simulink model "quadcoptersVerification"  (R2021b)
settings: Solver=ode4  StartTime=0.0  StopTime=inf  FixedStep=sampleTime_base  RelTol=1e-3
InitFcn:
  | initial_condition_sim;
values from neighbouring files (symbols this model uses):
  inertia = inertia'    [initial_condition_sim.m]
  kd_att = kd_att'    [initial_condition_sim.m]
  kp_att = kp_att'    [initial_condition_sim.m]
  lb_pos = lb_pos'    [initial_condition_sim.m]
  lb_vel = lb_vel'    [initial_condition_sim.m]
  motor_init_con = states_omeges(14:17,:)    [initial_condition_sim.m]
  number = 6    [initial_condition_sim.m]
  sampleTime_base = 0.01    [initial_condition_sim.m]
  sampleTime_control = 0.01    [initial_condition_sim.m]
  ub_pos = ub_pos'    [initial_condition_sim.m]
  ub_vel = ub_vel'    [initial_condition_sim.m]
  vehicle_int_con = states_omeges(1:13,:)    [initial_condition_sim.m]
undefined symbols (not defined in the file or in its folder): aMax_h, aMax_v, cd_filter_pos, cd_filter_vel, cm, ct, euler_max, get_array_slice, gravity, lenArm, mass, T_re, thrust_max, vMax_h, vMax_v, yaw_rate_max
libraries: dspindex x7, aerolibanimutils x1
settings Model: Creator=huangjialei  LastModifiedBy=huangjlei
settings SolverCC: AlgebraicLoopSolver=TrustRegion

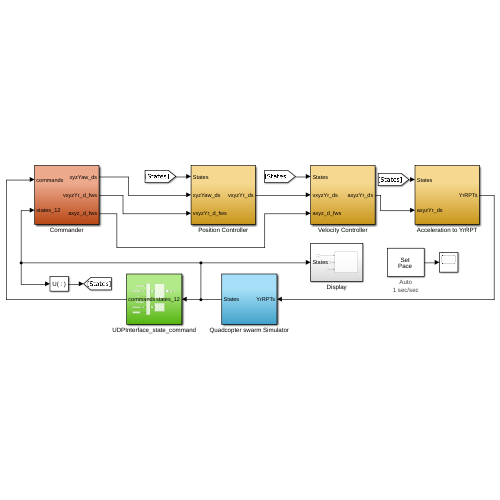
[thumbnail: Simulink's stored preview of the top-level diagram]
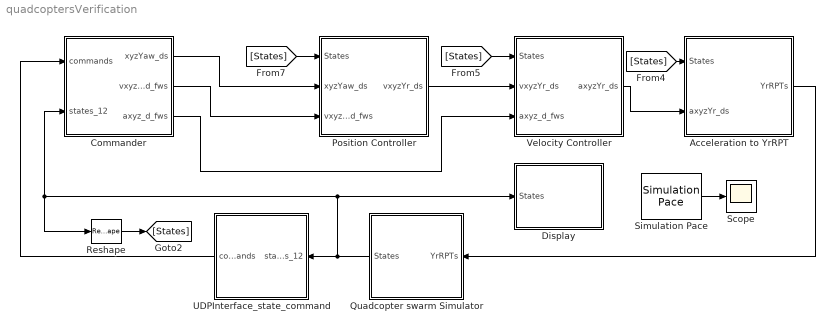
== system quadcoptersVerification ==
  Acceleration to YrRPT : Subsystem
  Commander : Subsystem
  Display : Subsystem
  Position Controller : Subsystem
  Quadcopter swarm Simulator : Subsystem
  Reshape : Reshape
  Scope : Scope
  Simulation Pace : aerolibanimutils/Simulation Pace  SimulationPace=1  SleepMode=Auto  OutputPaceError=on  SampleTime=sampleTime_base
  UDPInterface_state_command : Subsystem
  Velocity Controller : Subsystem
  wires:
  Commander/1(xyzYaw_ds) -> Position Controller/2(xyzYaw_ds)
  Commander/2(vxyzYr_d_fws) -> Position Controller/3(vxyzYr_d_fws)
  Simulation Pace/1 -> Scope/1
  Position Controller/1(vxyzYr_ds) -> Velocity Controller/2(vxyzYr_ds)
  Velocity Controller/1(axyzYr_ds) -> Acceleration to YrRPT/2(axyzYr_ds)
  Acceleration to YrRPT/1(YrRPTs) -> Quadcopter swarm Simulator/1(YrRPTs)
  [States] -> Acceleration to YrRPT/1(States)
  [States] -> Velocity Controller/1(States)
  [States] -> Position Controller/1(States)
  Commander/3(axyz_d_fws) -> Velocity Controller/3(axyz_d_fws)
  UDPInterface_state_command/1(commands) -> Commander/1(commands)
  Reshape/1 -> [States]
  Quadcopter swarm Simulator/1(States) -> UDPInterface_state_command/1(states_12), Commander/2(states_12), Reshape/1, Display/1(States)

== system quadcoptersVerification/Acceleration to YrRPT ==
  States : Inport
  axyzYr_ds : Inport  Port=2
  Selector : Selector  InputPortWidth=12*number  IndexOptions=Index vector (dialog)  Indices=10:12:12*number  OutputSizes=1
  Subsystem12 : Subsystem
  YrRPTs : Outport
  wires:
  States/1 -> Selector/1
  Selector/1 -> Subsystem12/2(yaws)
  Subsystem12/1(YrRPT) -> YrRPTs/1  "YrRPT"
  axyzYr_ds/1 -> Subsystem12/1(axyzYr_ds)

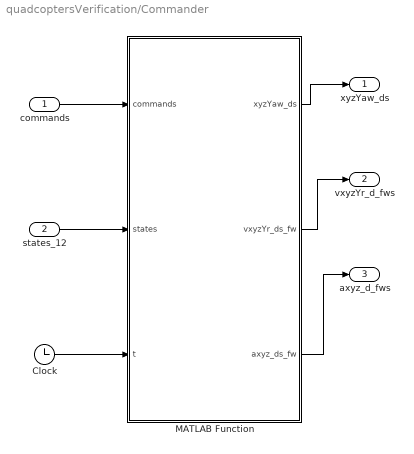
== system quadcoptersVerification/Commander ==
  commands : Inport
  states_12 : Inport  Port=2
  Clock : Clock
  MATLAB Function : MATLAB Function  TreatAsAtomicUnit=on  SystemSampleTime=sampleTime_control
  xyzYaw_ds : Outport
  vxyzYr_d_fws : Outport  Port=2
  axyz_d_fws : Outport  Port=3
  wires:
  Clock/1 -> MATLAB Function/3(t)
  MATLAB Function/2(vxyzYr_ds_fw) -> vxyzYr_d_fws/1
  MATLAB Function/1(xyzYaw_ds) -> xyzYaw_ds/1
  MATLAB Function/3(axyz_ds_fw) -> axyz_d_fws/1
  states_12/1 -> MATLAB Function/2(states)
  commands/1 -> MATLAB Function/1(commands)

== system quadcoptersVerification/Display ==
  States : Inport
  Clock : Clock
  Constant : Constant  Value=lenArm
  MATLAB Function : MATLAB Function  TreatAsAtomicUnit=on
  wires:
  Constant/1 -> MATLAB Function/2(lenArm)
  Clock/1 -> MATLAB Function/3(t)
  States/1 -> MATLAB Function/1(states)

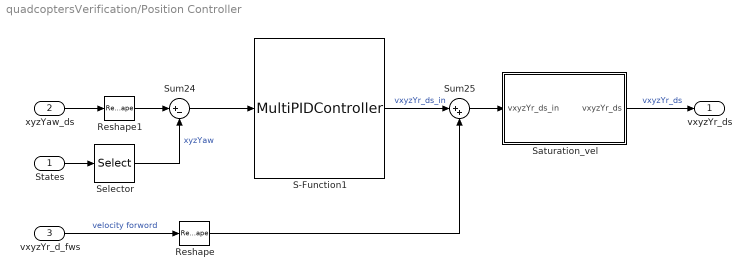
== system quadcoptersVerification/Position Controller ==
  States : Inport
  xyzYaw_ds : Inport  Port=2
  vxyzYr_d_fws : Inport  Port=3
  Reshape : Reshape
  Reshape1 : Reshape
  S-Function1 : S-Function  FunctionName=MultiPIDController  Parameters=sampleTime,number,width,enable_P,enable_I,enable_D,proportion,integral,derivative,c,enable_reset,lb,ub  SFunctionDeploymentMode=off  EnableBusSupport=off  mask{number=number, width=4, enable_P=on, enable_I=on, enable_D=on, proportion=[1,1,1,0], integral=[0,0,0,0], derivative=[0,0,3,0], c=cd_filter_pos, enable_reset=off, lb=lb_pos, ub=ub_pos, sampleTime=sampleTime_base}
      mask prompts: number "Number of input port"; width "Width of per input"; enable_P "Enable P"; enable_I "Enable I"; enable_D "Enable D"; c "Coefficient of low-pass filter in derivative part"; enable_reset "Rising edge reset of integral"; lb "Lower boundary of outputs"; ub "Upper boundary of outputs"; sampleTime "Sample time"
      mask Callback enable_P:
      | % disp(get_param(gcbh,'enable_P'))
      | % if strcmp(get_param(gcbh,'enable_P'), 'off')
      | %    disp(get_param(gcbh,'ParameterGroupVar'))
      | %
      | % end
  Saturation_vel : Subsystem
  Selector : Selector  InputPortWidth=12*number  IndexOptions=Index vector (dialog)  Indices=repmat([1,2,3,10],1,number) + reshape(repmat((0:number-1)*12,4,1),1,4*number)  OutputSizes=1
  Sum24 : Sum  Inputs=|+-
  Sum25 : Sum  Inputs=|++
  vxyzYr_ds : Outport
  wires:
  xyzYaw_ds/1 -> Reshape1/1
  States/1 -> Selector/1
  vxyzYr_d_fws/1 -> Reshape/1  "velocity forword"
  Sum24/1 -> S-Function1/1
  Selector/1 -> Sum24/2  "xyzYaw"
  S-Function1/1 -> Sum25/1  "vxyzYr_ds_in"
  Sum25/1 -> Saturation_vel/1(vxyzYr_ds_in)
  Saturation_vel/1(vxyzYr_ds) -> vxyzYr_ds/1  "vxyzYr_ds"
  Reshape/1 -> Sum25/2
  Reshape1/1 -> Sum24/1

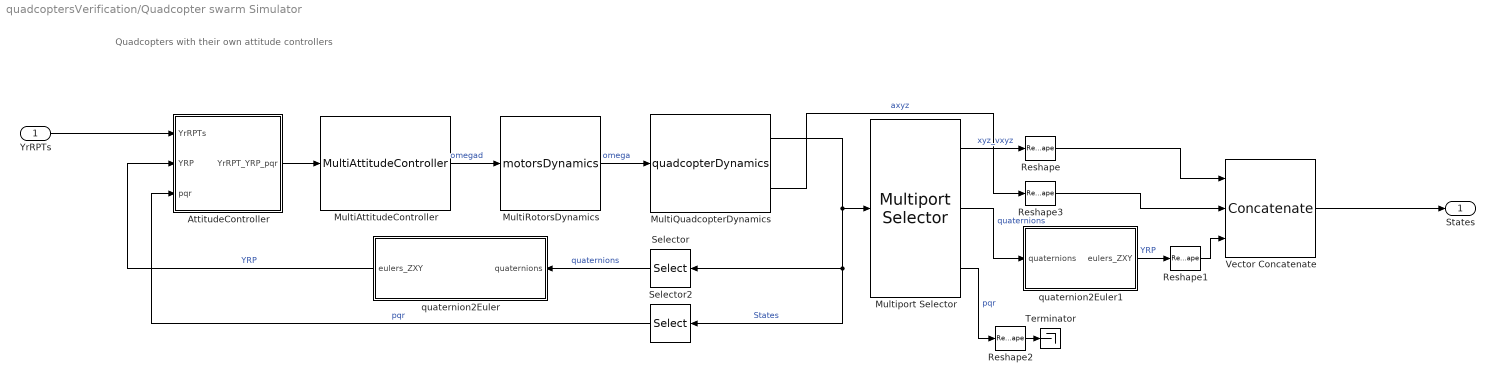
== system quadcoptersVerification/Quadcopter swarm Simulator ==
  note: Quadcopters with their own attitude controllers
  YrRPTs : Inport
  AttitudeController : Subsystem
  MultiAttitudeController : S-Function  FunctionName=MultiAttitudeController  Parameters=number_a,I_a,kp_a,kd_a,arm_length_a,ct_a,cm_a  SFunctionDeploymentMode=off  EnableBusSupport=off  mask{number_a=number+0, I_a=inertia, kp_a=kp_att, kd_a=kd_att, arm_length_a=lenArm, ct_a=ct, cm_a=cm}
      mask prompts: number_a "Number of quadcopters"; I_a "Moment of inertia"; kp_a "Coefficient of proportions"; kd_a "Coefficient of derivatives"; arm_length_a "Length of arm"; ct_a "Thrust coefficient of propeller"; cm_a "Moment coefficient of propeller"
      mask Display:
      | % number = get_param(gcbh,'number_a');
      | % for i = 1:str2num(number)
      | %    port_label('input', i, ['YrRPT_YRP_pqr',num2str(i)]);
      | % end
      | % for i = 1:str2num(number)
      | %    port_label('output', i, ['RPM_d',num2str(i)]);
      | % end
  MultiQuadcopterDynamics : S-Function  FunctionName=quadcopterDynamics  Parameters=number_q,mass_q,I_q,arm_length_q,ct_q,cm_q,conInit_q  SFunctionDeploymentMode=off  EnableBusSupport=off  mask{number_q=number+0, mass_q=mass, I_q=inertia, arm_length_q=lenArm, ct_q=ct, cm_q=cm, conInit_q=vehicle_int_con}
      mask prompts: number_q "Number of quadcopters"; mass_q "Mass"; I_q "Moment of inertia"; arm_length_q "Length of arm"; ct_q "Thrust coefficient of propeller"; cm_q "Moment coefficient of propeller"; conInit_q "Initial condition"
      mask Display:
      | number = get_param(gcbh,'number_q');
      | for i = 1:str2num(number)
      |    port_label('output', i, ['State',num2str(i)]);
      | end
      | for i = 1:str2num(number)
      |    port_label('input', i, ['RPM',num2str(i)]);
      | end
  MultiRotorsDynamics : S-Function  FunctionName=motorsDynamics  Parameters=number_m,K_m,conInit_m  SFunctionDeploymentMode=off  EnableBusSupport=off  mask{number_m=number+0, K_m=T_re, conInit_m=motor_init_con}
      mask prompts: number_m "Number of quadcopters"; K_m "Reciprocal of time constant"; conInit_m "Initial condition"
      mask Display:
      | number = get_param(gcbh,'number_m');
      | for i = 1:str2num(number)
      |    port_label('output', i, ['RPM',num2str(i)]);
      | end
      | for i = 1:str2num(number)
      |    port_label('input', i, ['RPM_d',num2str(i)]);
      | end
  Multiport Selector : dspindex/Multiport Selector  rowsOrCols=Rows  idxCellArray={ repmat(1:6,1,number) + reshape(repmat((0:number-1)*13,6,1),1,6*number),repmat(7:10,1,number) + reshape(repmat((0:number-1)*13,4,1),1,4*number), repmat(11:13,1,number) + reshape(repmat((0:number-1)*13,3,1),1,3*number)}  idxErrMode=Clip Index
  Reshape : Reshape  OutputDimensionality=Customize  OutputDimensions=[6,number]
  Reshape1 : Reshape  OutputDimensionality=Customize  OutputDimensions=[3,number]
  Reshape2 : Reshape  OutputDimensionality=Customize  OutputDimensions=[3,number]
  Reshape3 : Reshape  OutputDimensionality=Customize  OutputDimensions=[3,number]
  Selector : Selector  InputPortWidth=13*number  IndexOptions=Index vector (dialog)  Indices=repmat([7,8,9,10],1,number) + reshape(repmat((0:number-1)*13,4,1),1,4*number)  OutputSizes=1
  Selector2 : Selector  InputPortWidth=13*number  IndexOptions=Index vector (dialog)  Indices=repmat([11,12,13],1,number) + reshape(repmat((0:number-1)*13,3,1),1,3*number)  OutputSizes=1
  Terminator : Terminator
  Vector Concatenate : Concatenate  NumInputs=3  Mode=Multidimensional array
  quaternion2Euler : Subsystem
  quaternion2Euler1 : Subsystem
  States : Outport
  wires:
  YrRPTs/1 -> AttitudeController/1(YrRPTs)
  Selector/1 -> quaternion2Euler/1(quaternions)  "quaternions"
  quaternion2Euler/1(eulers_ZXY) -> AttitudeController/2(YRP)  "YRP"
  Selector2/1 -> AttitudeController/3(pqr)  "pqr"
  MultiAttitudeController/1 -> MultiRotorsDynamics/1  "omegad"
  MultiRotorsDynamics/1 -> MultiQuadcopterDynamics/1  "omega"
  MultiQuadcopterDynamics/1 -> Multiport Selector/1, Selector2/1, Selector/1  "States"
  Multiport Selector/2 -> quaternion2Euler1/1(quaternions)  "quaternions"
  Multiport Selector/1 -> Reshape/1  "xyz_vxyz"
  Reshape/1 -> Vector Concatenate/1
  quaternion2Euler1/1(eulers_ZXY) -> Reshape1/1  "YRP"
  Multiport Selector/3 -> Reshape2/1  "pqr"
  AttitudeController/1(YrRPT_YRP_pqr) -> MultiAttitudeController/1
  Vector Concatenate/1 -> States/1
  Reshape2/1 -> Terminator/1
  Reshape1/1 -> Vector Concatenate/3
  MultiQuadcopterDynamics/2 -> Reshape3/1  "axyz"
  Reshape3/1 -> Vector Concatenate/2

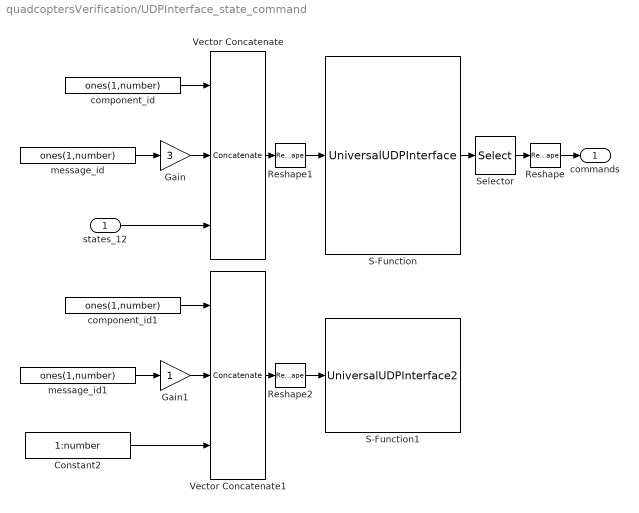
== system quadcoptersVerification/UDPInterface_state_command ==
  states_12 : Inport
  Constant2 : Constant  Value=1:number  VectorParams1D=off
  Gain : Gain  Gain=3
  Gain1 : Gain
  Reshape : Reshape  OutputDimensionality=Customize  OutputDimensions=[6,number]
  Reshape1 : Reshape
  Reshape2 : Reshape
  S-Function : S-Function  FunctionName=UniversalUDPInterface  Parameters=sampleTime,number,portTarget,portLocal,ipTarget,ipLocal,flagSend,flagRecv,inputPortWidth,outputPortWidth  SFunctionDeploymentMode=off  EnableBusSupport=off  mask{number=number, ipLocal=127.0.0.1, ipTarget=ones(1,number)*1, portTarget=20999, portLocal=21001, flagSend=on, flagRecv=on, inputPortWidth=14, outputPortWidth=9, sampleTime=sampleTime_control}
      mask prompts: number "Number of vehicles"; ipLocal "Local ip"; ipTarget "Target ip"; portTarget "Start port of target"; portLocal "Start port of local"; flagSend "Enable sender"; flagRecv "Enable receiver"; inputPortWidth "Width of input port"; outputPortWidth "Width of output port"; sampleTime "Sample time"
      mask help:
      | input port: componentId, messageId, msgData[0], msgData[1], ...
      | output port: systemId, numSequence, timeStamp,msgData[0], msgData[1], ...
  S-Function1 : S-Function  FunctionName=UniversalUDPInterface2  Parameters=sampleTime,number,portTarget,portLocal,ipTarget,ipLocal,flagSend,flagRecv,inputPortWidth,outputPortWidth  SFunctionDeploymentMode=off  EnableBusSupport=off  mask{number=number, ipLocal=127.0.0.1, ipTarget=ones(1,number)*1, portTarget=19999, portLocal=22001, flagSend=on, flagRecv=off, inputPortWidth=3, outputPortWidth=9, sampleTime=sampleTime_control}
      mask prompts: number "Number of vehicles"; ipLocal "Local ip"; ipTarget "Target ip"; portTarget "Start port of target"; portLocal "Start port of local"; flagSend "Enable sender"; flagRecv "Enable receiver"; inputPortWidth "Width of input port"; outputPortWidth "Width of output port"; sampleTime "Sample time"
      mask help:
      | input port: componentId, messageId, msgData[0], msgData[1], ...
      | output port: systemId, numSequence, timeStamp,msgData[0], msgData[1], ...
  Selector : Selector  InputPortWidth=9*number  IndexOptions=Index vector (dialog)  Indices=get_array_slice(4:9, number, 9)  OutputSizes=1
  Vector Concatenate : Concatenate  NumInputs=3  Mode=Multidimensional array
  Vector Concatenate1 : Concatenate  NumInputs=3  Mode=Multidimensional array
  component_id : Constant  Value=ones(1,number)  VectorParams1D=off
  component_id1 : Constant  Value=ones(1,number)  VectorParams1D=off
  message_id : Constant  Value=ones(1,number)  VectorParams1D=off
  message_id1 : Constant  Value=ones(1,number)  VectorParams1D=off
  commands : Outport
  wires:
  Vector Concatenate/1 -> Reshape1/1
  Reshape1/1 -> S-Function/1
  component_id/1 -> Vector Concatenate/1
  message_id/1 -> Gain/1
  Gain/1 -> Vector Concatenate/2
  S-Function/1 -> Selector/1
  Gain1/1 -> Vector Concatenate1/2
  message_id1/1 -> Gain1/1
  Constant2/1 -> Vector Concatenate1/3
  component_id1/1 -> Vector Concatenate1/1
  Reshape2/1 -> S-Function1/1
  Vector Concatenate1/1 -> Reshape2/1
  states_12/1 -> Vector Concatenate/3
  Selector/1 -> Reshape/1
  Reshape/1 -> commands/1

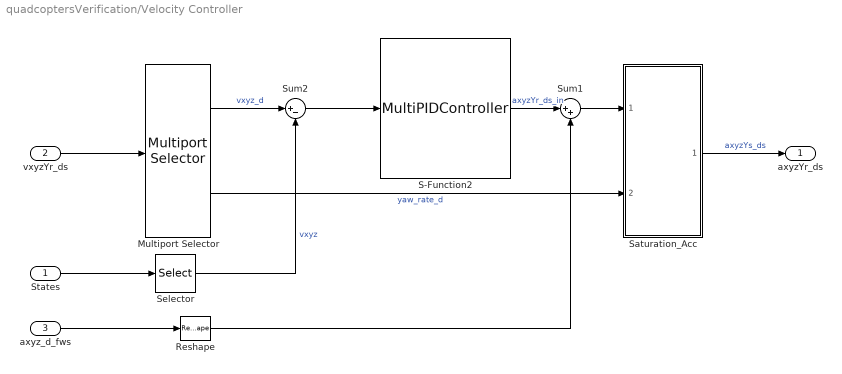
== system quadcoptersVerification/Velocity Controller ==
  States : Inport
  vxyzYr_ds : Inport  Port=2
  axyz_d_fws : Inport  Port=3
  Multiport Selector : dspindex/Multiport Selector  rowsOrCols=Rows  idxCellArray={ repmat([1,2,3],1,number) + reshape(repmat((0:number-1)*4,3,1),1,3*number),4:4:4*number}  idxErrMode=Clip Index
  Reshape : Reshape
  S-Function2 : S-Function  FunctionName=MultiPIDController  Parameters=sampleTime,number,width,enable_P,enable_I,enable_D,proportion,integral,derivative,c,enable_reset,lb,ub  SFunctionDeploymentMode=off  EnableBusSupport=off  mask{number=number+0, width=3, enable_P=on, enable_I=on, enable_D=on, proportion=[1.2,1.2,1], integral=[2,2,0.8], derivative=[0.3,0.3,0], c=cd_filter_vel, enable_reset=off, lb=lb_vel, ub=ub_vel, sampleTime=sampleTime_base}
      mask prompts: number "Number of input port"; width "Width of per input"; enable_P "Enable P"; enable_I "Enable I"; enable_D "Enable D"; c "Coefficient of low-pass filter in derivative part"; enable_reset "Rising edge reset of integral"; lb "Lower boundary of outputs"; ub "Upper boundary of outputs"; sampleTime "Sample time"
      mask Callback enable_P:
      | % disp(get_param(gcbh,'enable_P'))
      | % if strcmp(get_param(gcbh,'enable_P'), 'off')
      | %    disp(get_param(gcbh,'ParameterGroupVar'))
      | %
      | % end
  Saturation_Acc : Subsystem
  Selector : Selector  InputPortWidth=12*number  IndexOptions=Index vector (dialog)  Indices=repmat([4,5,6],1,number) + reshape(repmat((0:number-1)*12,3,1),1,3*number)  OutputSizes=1
  Sum1 : Sum  Inputs=|++
  Sum2 : Sum  Inputs=|+-
  axyzYr_ds : Outport
  wires:
  States/1 -> Selector/1
  Selector/1 -> Sum2/2  "vxyz"
  Sum2/1 -> S-Function2/1
  Multiport Selector/1 -> Sum2/1  "vxyz_d"
  Multiport Selector/2 -> Saturation_Acc/2(yaw_rates)  "yaw_rate_d"
  vxyzYr_ds/1 -> Multiport Selector/1
  Saturation_Acc/1(axyzYr_ds) -> axyzYr_ds/1  "axyzYs_ds"
  S-Function2/1 -> Sum1/1  "axyzYr_ds_in"
  Sum1/1 -> Saturation_Acc/1(axyz_d_in)
  axyz_d_fws/1 -> Reshape/1
  Reshape/1 -> Sum1/2

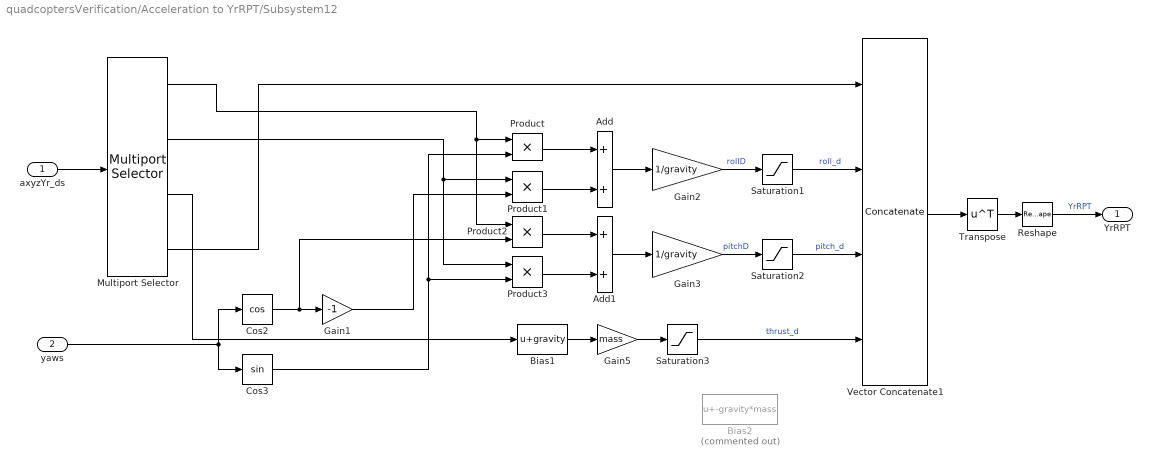
== system quadcoptersVerification/Acceleration to YrRPT/Subsystem12 ==
  axyzYr_ds : Inport
  yaws : Inport  Port=2
  Add : Sum
  Add1 : Sum
  Bias1 : Bias  Bias=gravity
  Bias2 : Bias  Commented=on  Bias=-gravity*mass
  Cos2 : Trigonometry  Operator=cos
  Cos3 : Trigonometry
  Gain1 : Gain  Gain=-1
  Gain2 : Gain  Gain=1/gravity
  Gain3 : Gain  Gain=1/gravity
  Gain5 : Gain  Gain=mass
  Multiport Selector : dspindex/Multiport Selector  rowsOrCols=Rows  idxCellArray={ 1:4:4*number,2:4:4*number, 3:4:4*number,4:4:4*number}  idxErrMode=Clip Index
  Product{,1..3} (4 alike) : Product
  Reshape : Reshape
  Saturation1 : Saturate  UpperLimit=euler_max  LowerLimit=-euler_max
  Saturation2 : Saturate  UpperLimit=euler_max  LowerLimit=-euler_max
  Saturation3 : Saturate  UpperLimit=thrust_max  LowerLimit=0
  Transpose : Math  Operator=transpose  SaturateOnIntegerOverflow=on
  Vector Concatenate1 : Concatenate  NumInputs=4  Mode=Multidimensional array  ConcatenateDimension=2
  YrRPT : Outport
  wires:
  Saturation3/1 -> Vector Concatenate1/4  "thrust_d"
  Saturation2/1 -> Vector Concatenate1/3  "pitch_d"
  Saturation1/1 -> Vector Concatenate1/2  "roll_d"
  Gain5/1 -> Saturation3/1
  Multiport Selector/4 -> Vector Concatenate1/1
  Reshape/1 -> YrRPT/1  "YrRPT"
  Gain2/1 -> Saturation1/1  "rollD"
  Add/1 -> Gain2/1
  Multiport Selector/1 -> Product/1, Product2/1
  Gain1/1 -> Product1/2
  Product/1 -> Add/1
  axyzYr_ds/1 -> Multiport Selector/1
  Product3/1 -> Add1/2
  Cos2/1 -> Gain1/1, Product2/2
  Product1/1 -> Add/2
  Multiport Selector/3 -> Bias1/1
  Gain3/1 -> Saturation2/1  "pitchD"
  Product2/1 -> Add1/1
  Multiport Selector/2 -> Product1/1, Product3/1
  Cos3/1 -> Product3/2, Product/2
  Add1/1 -> Gain3/1
  yaws/1 -> Cos2/1, Cos3/1
  Bias1/1 -> Gain5/1
  Vector Concatenate1/1 -> Transpose/1
  Transpose/1 -> Reshape/1

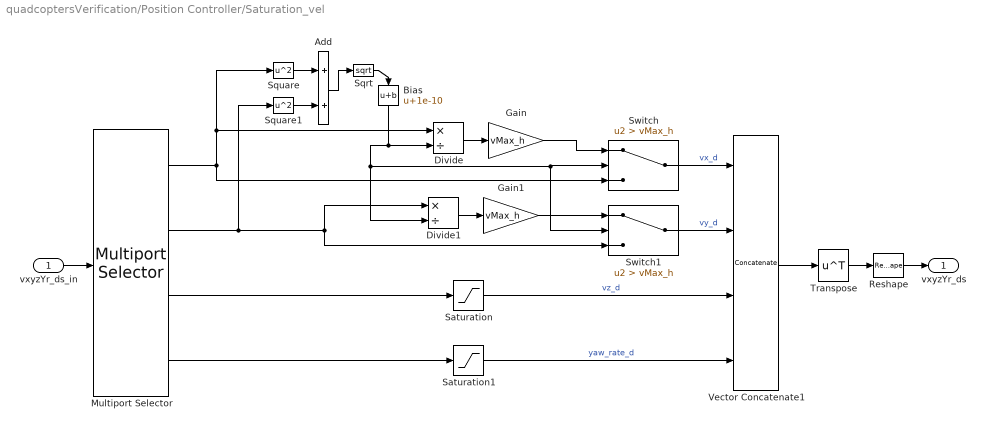
== system quadcoptersVerification/Position Controller/Saturation_vel ==
  vxyzYr_ds_in : Inport
  Add : Sum
  Bias : Bias  Bias=1e-10
  Divide : Product  Inputs=*/
  Divide1 : Product  Inputs=*/
  Gain : Gain  Gain=vMax_h
  Gain1 : Gain  Gain=vMax_h
  Multiport Selector : dspindex/Multiport Selector  rowsOrCols=Rows  idxCellArray={ 1:4:4*number,2:4:4*number, 3:4:4*number, 4:4:4*number }  idxErrMode=Clip Index
  Reshape : Reshape
  Saturation : Saturate  UpperLimit=vMax_v  LowerLimit=-vMax_v
  Saturation1 : Saturate  UpperLimit=yaw_rate_max  LowerLimit=-yaw_rate_max
  Sqrt : Sqrt  SaturateOnIntegerOverflow=on
  Square : Math  Operator=square  SaturateOnIntegerOverflow=on
  Square1 : Math  Operator=square  SaturateOnIntegerOverflow=on
  Switch : Switch  Criteria=u2 > Threshold  Threshold=vMax_h
  Switch1 : Switch  Criteria=u2 > Threshold  Threshold=vMax_h
  Transpose : Math  Operator=transpose  SaturateOnIntegerOverflow=on
  Vector Concatenate1 : Concatenate  NumInputs=4  Mode=Multidimensional array  ConcatenateDimension=2
  vxyzYr_ds : Outport
  wires:
  Switch/1 -> Vector Concatenate1/1  "vx_d"
  Multiport Selector/3 -> Saturation/1
  Gain/1 -> Switch/1
  Divide/1 -> Gain/1
  Multiport Selector/1 -> Square/1, Divide/1, Switch/3
  Add/1 -> Sqrt/1
  Square1/1 -> Add/2
  Square/1 -> Add/1
  vxyzYr_ds_in/1 -> Multiport Selector/1
  Multiport Selector/4 -> Saturation1/1
  Saturation1/1 -> Vector Concatenate1/4  "yaw_rate_d"
  Saturation/1 -> Vector Concatenate1/3  "vz_d"
  Sqrt/1 -> Bias/1
  Multiport Selector/2 -> Divide1/1, Switch1/3, Square1/1
  Divide1/1 -> Gain1/1
  Gain1/1 -> Switch1/1
  Switch1/1 -> Vector Concatenate1/2  "vy_d"
  Vector Concatenate1/1 -> Transpose/1
  Transpose/1 -> Reshape/1
  Reshape/1 -> vxyzYr_ds/1
  Bias/1 -> Divide/2, Divide1/2, Switch/2, Switch1/2

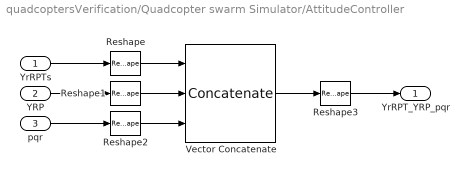
== system quadcoptersVerification/Quadcopter swarm Simulator/AttitudeController ==
  YrRPTs : Inport
  YRP : Inport  Port=2
  pqr : Inport  Port=3
  Reshape : Reshape  OutputDimensionality=Customize  OutputDimensions=[4,number]
  Reshape1 : Reshape  OutputDimensionality=Customize  OutputDimensions=[3,number]
  Reshape2 : Reshape  OutputDimensionality=Customize  OutputDimensions=[3,number]
  Reshape3 : Reshape
  Vector Concatenate : Concatenate  NumInputs=3  Mode=Multidimensional array
  YrRPT_YRP_pqr : Outport
  wires:
  YrRPTs/1 -> Reshape/1
  YRP/1 -> Reshape1/1
  pqr/1 -> Reshape2/1
  Reshape/1 -> Vector Concatenate/1
  Reshape1/1 -> Vector Concatenate/2
  Reshape2/1 -> Vector Concatenate/3
  Vector Concatenate/1 -> Reshape3/1
  Reshape3/1 -> YrRPT_YRP_pqr/1

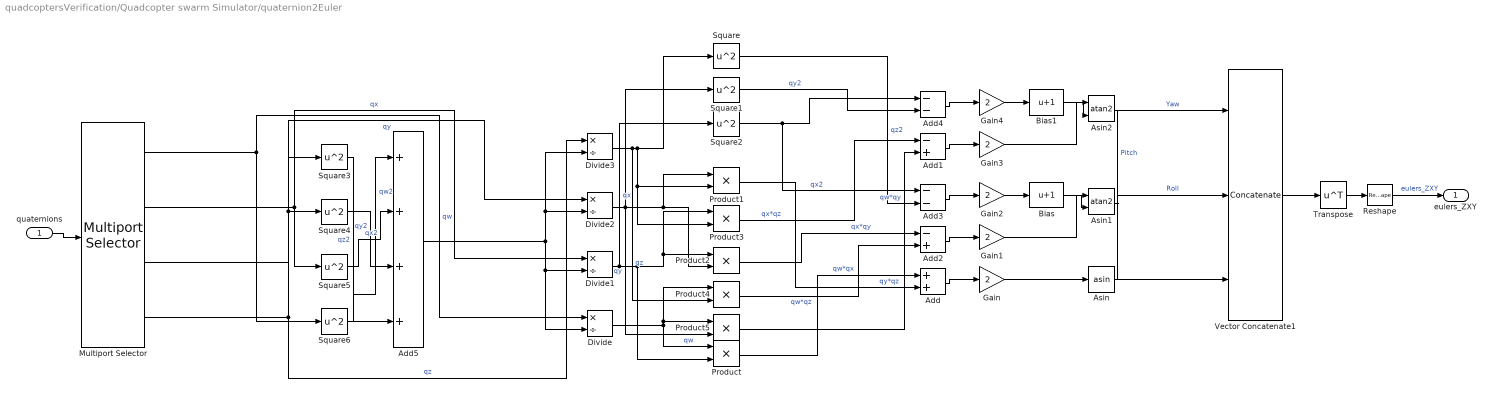
== system quadcoptersVerification/Quadcopter swarm Simulator/quaternion2Euler ==
  quaternions : Inport
  Add : Sum
  Add1 : Sum  Inputs=-+
  Add2 : Sum  Inputs=-+
  Add3 : Sum  Inputs=--
  Add4 : Sum  Inputs=--
  Add5 : Sum  Inputs=++++
  Asin : Trigonometry  Operator=asin
  Asin1 : Trigonometry  Operator=atan2
  Asin2 : Trigonometry  Operator=atan2
  Bias : Bias  Bias=1
  Bias1 : Bias  Bias=1
  Divide{,1..3} (4 alike) : Product  Inputs=*/
  Gain{,1..4} (5 alike) : Gain  Gain=2
  Multiport Selector : dspindex/Multiport Selector  rowsOrCols=Rows  idxCellArray={ 1:4:4*number,2:4:4*number, 3:4:4*number, 4:4:4*number }  idxErrMode=Clip Index
  Product{,1..5} (6 alike) : Product
  Reshape : Reshape
  Square{,1..6} (7 alike) : Math  Operator=square  SaturateOnIntegerOverflow=on
  Transpose : Math  Operator=transpose  SaturateOnIntegerOverflow=on
  Vector Concatenate1 : Concatenate  NumInputs=3  Mode=Multidimensional array  ConcatenateDimension=2
  eulers_ZXY : Outport
  wires:
  Multiport Selector/1 -> Divide/1, Square6/1  "qw"
  Add5/1 -> Divide1/2, Divide/2, Divide3/2, Divide2/2
  Square4/1 -> Add5/3  "qy2"
  Add/1 -> Gain/1
  quaternions/1 -> Multiport Selector/1
  Multiport Selector/4 -> Divide3/1, Square3/1  "qz"
  Product/1 -> Add/1  "qw*qx"
  Divide2/1 -> Product1/1, Product2/2, Product5/2, Square1/1  "qy"
  Reshape/1 -> eulers_ZXY/1  "eulers_ZXY"
  Product1/1 -> Add/2  "qy*qz"
  Divide1/1 -> Product3/1, Product2/1, Product/2, Square2/1  "qx"
  Square6/1 -> Add5/1  "qw2"
  Asin/1 -> Vector Concatenate1/2  "Roll"
  Square5/1 -> Add5/2  "qx2"
  Asin1/1 -> Vector Concatenate1/1  "Yaw"
  Product4/1 -> Add2/2  "qw*qz"
  Multiport Selector/2 -> Square5/1, Divide1/1  "qx"
  Product2/1 -> Add2/1  "qx*qy"
  Product3/1 -> Add1/1  "qx*qz"
  Gain/1 -> Asin/1
  Divide/1 -> Product5/1, Product4/1, Product/1  "qw"
  Gain3/1 -> Asin2/1
  Gain4/1 -> Bias1/1
  Divide3/1 -> Product3/2, Product1/2, Square/1, Product4/2  "qz"
  Square/1 -> Add3/2  "qz2"
  Add1/1 -> Gain3/1
  Bias1/1 -> Asin2/2
  Add2/1 -> Gain1/1
  Add4/1 -> Gain4/1
  Asin2/1 -> Vector Concatenate1/3  "Pitch"
  Multiport Selector/3 -> Divide2/1, Square4/1  "qy"
  Square3/1 -> Add5/4  "qz2"
  Square2/1 -> Add3/1, Add4/1  "qx2"
  Square1/1 -> Add4/2  "qy2"
  Vector Concatenate1/1 -> Transpose/1
  Bias/1 -> Asin1/2
  Gain2/1 -> Bias/1
  Add3/1 -> Gain2/1
  Gain1/1 -> Asin1/1
  Transpose/1 -> Reshape/1
  Product5/1 -> Add1/2  "qw*qy"

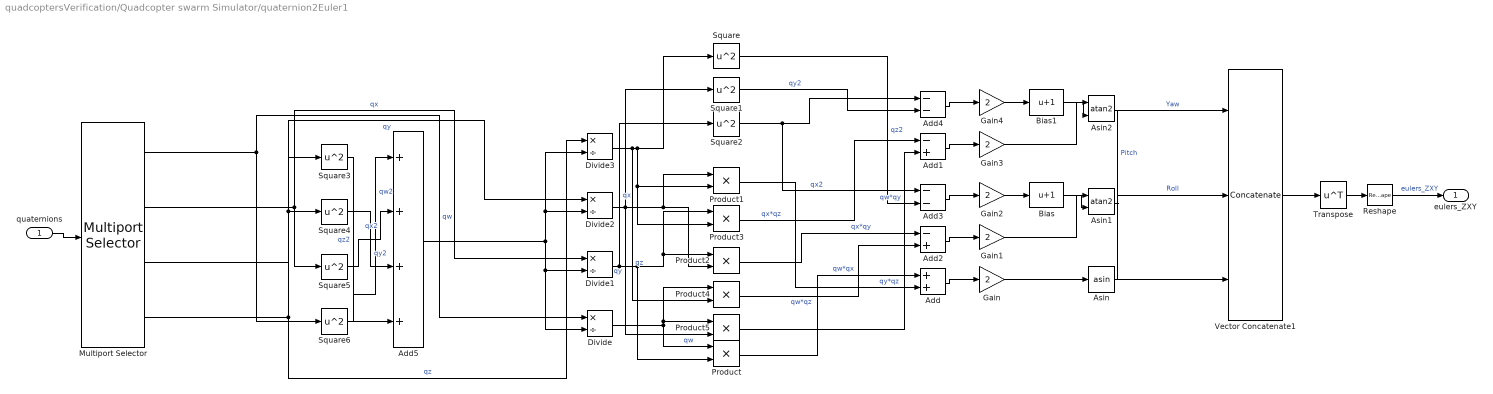
== system quadcoptersVerification/Quadcopter swarm Simulator/quaternion2Euler1 ==
  quaternions : Inport
  Add : Sum
  Add1 : Sum  Inputs=-+
  Add2 : Sum  Inputs=-+
  Add3 : Sum  Inputs=--
  Add4 : Sum  Inputs=--
  Add5 : Sum  Inputs=++++
  Asin : Trigonometry  Operator=asin
  Asin1 : Trigonometry  Operator=atan2
  Asin2 : Trigonometry  Operator=atan2
  Bias : Bias  Bias=1
  Bias1 : Bias  Bias=1
  Divide{,1..3} (4 alike) : Product  Inputs=*/
  Gain{,1..4} (5 alike) : Gain  Gain=2
  Multiport Selector : dspindex/Multiport Selector  rowsOrCols=Rows  idxCellArray={ 1:4:4*number,2:4:4*number, 3:4:4*number, 4:4:4*number }  idxErrMode=Clip Index
  Product{,1..5} (6 alike) : Product
  Reshape : Reshape
  Square{,1..6} (7 alike) : Math  Operator=square  SaturateOnIntegerOverflow=on
  Transpose : Math  Operator=transpose  SaturateOnIntegerOverflow=on
  Vector Concatenate1 : Concatenate  NumInputs=3  Mode=Multidimensional array  ConcatenateDimension=2
  eulers_ZXY : Outport
  wires:
  Product5/1 -> Add1/2  "qw*qy"
  Transpose/1 -> Reshape/1
  Gain1/1 -> Asin1/1
  Add3/1 -> Gain2/1
  Gain2/1 -> Bias/1
  Bias/1 -> Asin1/2
  Vector Concatenate1/1 -> Transpose/1
  Square1/1 -> Add4/2  "qy2"
  Square2/1 -> Add4/1, Add3/1  "qx2"
  Square3/1 -> Add5/4  "qz2"
  Multiport Selector/3 -> Square4/1, Divide2/1  "qy"
  Asin2/1 -> Vector Concatenate1/3  "Pitch"
  Add4/1 -> Gain4/1
  Add2/1 -> Gain1/1
  Bias1/1 -> Asin2/2
  Add1/1 -> Gain3/1
  Square/1 -> Add3/2  "qz2"
  Divide3/1 -> Product4/2, Square/1, Product1/2, Product3/2  "qz"
  Gain4/1 -> Bias1/1
  Gain3/1 -> Asin2/1
  Divide/1 -> Product/1, Product4/1, Product5/1  "qw"
  Gain/1 -> Asin/1
  Product3/1 -> Add1/1  "qx*qz"
  Product2/1 -> Add2/1  "qx*qy"
  Multiport Selector/2 -> Divide1/1, Square5/1  "qx"
  Product4/1 -> Add2/2  "qw*qz"
  Asin1/1 -> Vector Concatenate1/1  "Yaw"
  Square5/1 -> Add5/2  "qx2"
  Asin/1 -> Vector Concatenate1/2  "Roll"
  Square6/1 -> Add5/1  "qw2"
  Divide1/1 -> Square2/1, Product/2, Product2/1, Product3/1  "qx"
  Product1/1 -> Add/2  "qy*qz"
  Reshape/1 -> eulers_ZXY/1  "eulers_ZXY"
  Divide2/1 -> Square1/1, Product5/2, Product2/2, Product1/1  "qy"
  Product/1 -> Add/1  "qw*qx"
  Multiport Selector/4 -> Square3/1, Divide3/1  "qz"
  quaternions/1 -> Multiport Selector/1
  Add/1 -> Gain/1
  Square4/1 -> Add5/3  "qy2"
  Add5/1 -> Divide2/2, Divide3/2, Divide/2, Divide1/2
  Multiport Selector/1 -> Square6/1, Divide/1  "qw"

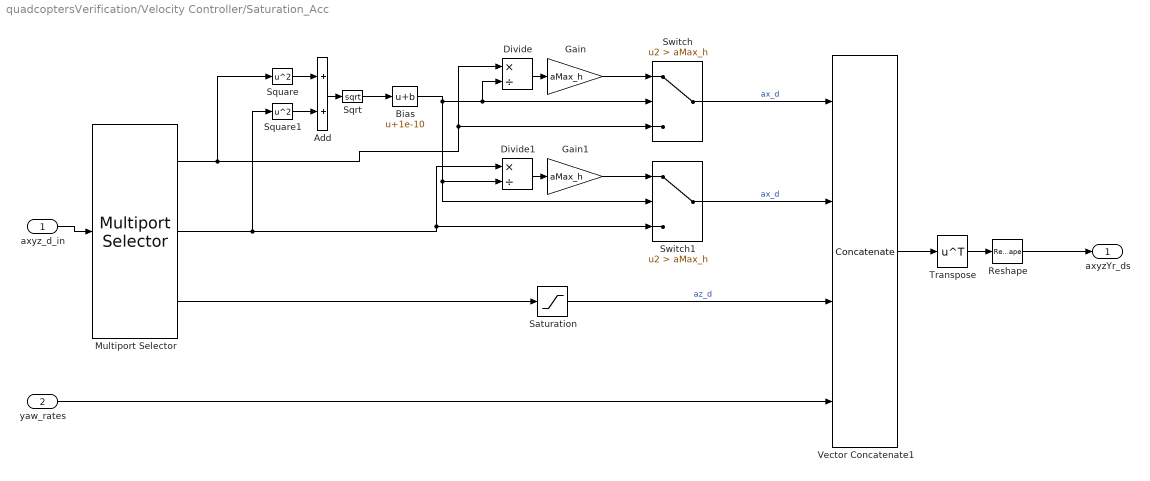
== system quadcoptersVerification/Velocity Controller/Saturation_Acc ==
  axyz_d_in : Inport
  yaw_rates : Inport  Port=2
  Add : Sum
  Bias : Bias  Bias=1e-10
  Divide : Product  Inputs=*/
  Divide1 : Product  Inputs=*/
  Gain : Gain  Gain=aMax_h
  Gain1 : Gain  Gain=aMax_h
  Multiport Selector : dspindex/Multiport Selector  rowsOrCols=Rows  idxCellArray={ 1:3:3*number,2:3:3*number, 3:3:3*number}  idxErrMode=Clip Index
  Reshape : Reshape
  Saturation : Saturate  UpperLimit=aMax_v  LowerLimit=-aMax_v
  Sqrt : Sqrt  SaturateOnIntegerOverflow=on
  Square : Math  Operator=square  SaturateOnIntegerOverflow=on
  Square1 : Math  Operator=square  SaturateOnIntegerOverflow=on
  Switch : Switch  Criteria=u2 > Threshold  Threshold=aMax_h
  Switch1 : Switch  Criteria=u2 > Threshold  Threshold=aMax_h
  Transpose : Math  Operator=transpose  SaturateOnIntegerOverflow=on
  Vector Concatenate1 : Concatenate  NumInputs=4  Mode=Multidimensional array  ConcatenateDimension=2
  axyzYr_ds : Outport
  wires:
  Switch/1 -> Vector Concatenate1/1  "ax_d"
  Saturation/1 -> Vector Concatenate1/3  "az_d"
  Reshape/1 -> axyzYr_ds/1
  Multiport Selector/3 -> Saturation/1
  Gain/1 -> Switch/1
  Divide/1 -> Gain/1
  Multiport Selector/1 -> Switch/3, Divide/1, Square/1
  Add/1 -> Sqrt/1
  Square1/1 -> Add/2
  Square/1 -> Add/1
  axyz_d_in/1 -> Multiport Selector/1
  Sqrt/1 -> Bias/1
  Multiport Selector/2 -> Switch1/3, Divide1/1, Square1/1
  Divide1/1 -> Gain1/1
  Gain1/1 -> Switch1/1
  Switch1/1 -> Vector Concatenate1/2  "ax_d"
  Transpose/1 -> Reshape/1
  Vector Concatenate1/1 -> Transpose/1
  yaw_rates/1 -> Vector Concatenate1/4
  Bias/1 -> Switch/2, Divide/2, Switch1/2, Divide1/2

== matlab function quadcoptersVerification/Commander/MATLAB Function ==
  settings: updateMethod=DISCRETE
  data: commands input; xyzYaw_ds output; states input; t input; vxyzYr_ds_fw output; axyz_ds_fw output
function [xyzYaw_ds, vxyzYr_ds_fw, axyz_ds_fw] = commander(commands, states,t)
persistent states_save  message_Ids_former t_start_Circle t_trigger v_save vx_save vy_save
number = size(states,2);
if isempty(states_save) || t < 0.1
    states_save = states;
    message_Ids_former = zeros(1,number)-1;
end
xyz_s = states(1:3,:);
% vxyz_s = states(4:6,:);
% axyz_s = states(7:9,:);
yrp_s = states(10:12,:);

xyzYaw_ds = [xyz_s;yrp_s(1,:)];
vxyzYr_ds_fw = zeros(4,number);
axyz_ds_fw   = zeros(3,number);



component_ids = commands(1,:);
message_ids = commands(2,:);
msgs = commands(3:6,:);

COMMAND_TYPE = 0;

Arming = 1;
Takeoff = 2;
Hover = 3;
Land = 4;
Position_control = 5;
Velocity_control = 6;
Velocity_horizontal_control = 7;
Acceleration_control = 8;

for id = 1:number
    component_id = component_ids(id);
    if component_id == COMMAND_TYPE
        message_id = message_ids(id);
        message_id_former = message_Ids_former(id);
        msg = msgs(:,id);
        switch message_id
            case Takeoff
                if message_id_former ~= message_id
%                     str = sprintf("UAV %d takeoff.",id);
%                     disp(str);
%                     disp(str);
                    fprintf("UAV %d takeoff.\n",int16(id));
                    states_save(:,id) = states(:,id);
                end
                xyzYaw_ds(:,id) = states_save([1,2,3,10],id);
                xyzYaw_ds(3,id) = msg(1);
            case Hover
                if message_id_former ~= message_id
%                     disp(['UAV ',num2str(id),' hover.']);
                    states_save(:,id) = states(:,id);
                end
                xyzYaw_ds(:,id) = states_save([1,2,3,10],id);
            case Land
                if message_id_former ~= message_id
%                     disp(['UAV ',num2str(id),' land.']);
                    states_save(:,id) = states(:,id);
                end
                xyzYaw_ds(:,id) = states_save([1,2,3,10],id);
                xyzYaw_ds(3,id) = msg(1);
            case Position_control
                if message_id_former ~= message_id
%                     disp(['UAV ',num2str(id),' position control.']);
                end
                xyzYaw_ds(:,id) = msg;
            case Velocity_control
                if message_id_former ~= message_id
%                     disp(['UAV ',num2str(id),' velocity control.']);
                end
                vxyzYr_ds_fw(:,id) = msg;
            case Velocity_horizontal_control
                if message_id_former ~= message_id
%                     disp(['UAV ',num2str(id),' velocity horizontal control.']);
                end
                vxyzYr_ds_fw([1,2,4],id) = msg([1,2,4]);
                xyzYaw_ds(3,id) = msg(3);
            case Acceleration_control
                if message_id_former ~= message_id
%                     disp(['UAV ',num2str(id),' acceleration control.']);
                end
                axyz_ds_fw(:,id) = msg(1:3);
        end
        message_Ids_former(id) = message_id;
    end
end

== matlab function quadcoptersVerification/Display/MATLAB Function ==
  settings: updateMethod=DISCRETE
  data: states input; lenArm input; t input
function fcn(states,lenArm, t)
persistent t_last count
figure(1)
if isempty(t_last)
    t_last = 0;
    count = 1;
    myFigure = figure(1);
    cla(myFigure);
    hold on
    grid on
    box on
    axis equal
    view([-35,35]);
    xlim([-4,4]);
    ylim([-4,4]);
    zlim([0,3]);
    xlabel('X Position (m)')
    ylabel('Y Position (m)')
    plotMultiQuadcopters(myFigure,states,lenArm);
end
if t - t_last > 0.5
    myFigure = figure(1);
    cla(myFigure);
    plotMultiQuadcopters(myFigure,states,lenArm);
%     xlim([-2,2]);
%     ylim([-3.5,3]);
%     zlim([0,2]);
    t_last = t;
end
count = count + 1;
